simulink model "quat_difference"  (R2024a)
settings: Solver=VariableStepAuto  StartTime=0.0  StopTime=10.0  RelTol=1e-3
libraries: sharedtransform x5, aerolibutil x1
settings Model: Creator=bemran  LastModifiedBy=bemran

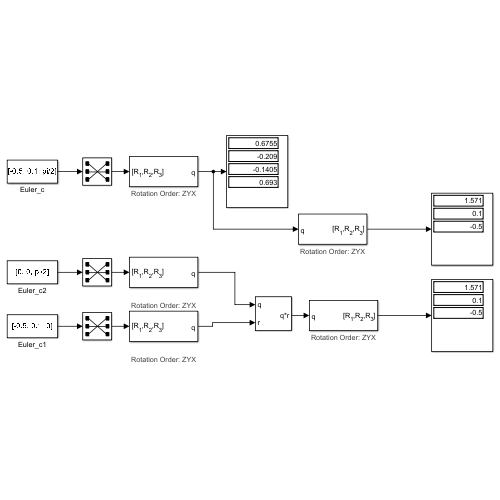
[thumbnail: Simulink's stored preview of the top-level diagram]
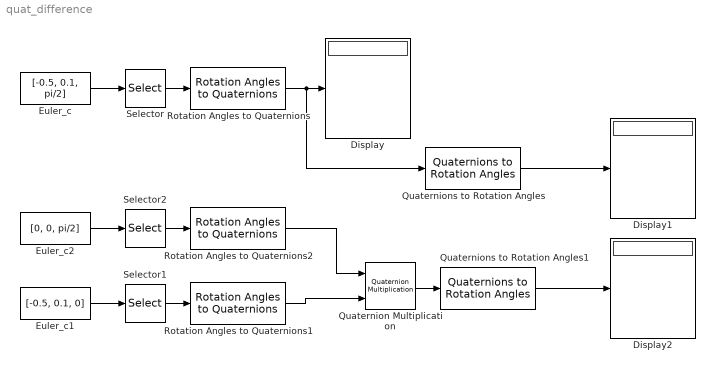
== system quat_difference ==
  Display : Display
  Display1 : Display
  Display2 : Display
  Euler_c : Constant  Value=[-0.5, 0.1, pi/2]
  Euler_c1 : Constant  Value=[-0.5, 0.1, 0]
  Euler_c2 : Constant  Value=[0, 0, pi/2]
  Quaternion Multiplication : aerolibutil/Quaternion Multiplication
  Quaternions to Rotation Angles : sharedtransform/Quaternions to Rotation Angles  rotationOrder=ZYX  aMode=aMode
  Quaternions to Rotation Angles1 : sharedtransform/Quaternions to Rotation Angles  rotationOrder=ZYX  aMode=aMode
  Rotation Angles to Quaternions : sharedtransform/Rotation Angles to Quaternions  rotationOrder=ZYX  aMode=aMode
  Rotation Angles to Quaternions1 : sharedtransform/Rotation Angles to Quaternions  rotationOrder=ZYX  aMode=aMode
  Rotation Angles to Quaternions2 : sharedtransform/Rotation Angles to Quaternions  rotationOrder=ZYX  aMode=aMode
  Selector : Selector  InputPortWidth=3  IndexOptions=Index vector (dialog)  Indices=[3 2 1]  OutputSizes=1
  Selector1 : Selector  InputPortWidth=3  IndexOptions=Index vector (dialog)  Indices=[3 2 1]  OutputSizes=1
  Selector2 : Selector  InputPortWidth=3  IndexOptions=Index vector (dialog)  Indices=[3 2 1]  OutputSizes=1
  wires:
  Selector/1 -> Rotation Angles to Quaternions/1
  Euler_c/1 -> Selector/1
  Rotation Angles to Quaternions/1 -> Quaternions to Rotation Angles/1, Display/1
  Euler_c1/1 -> Selector1/1
  Selector1/1 -> Rotation Angles to Quaternions1/1
  Selector2/1 -> Rotation Angles to Quaternions2/1
  Euler_c2/1 -> Selector2/1
  Rotation Angles to Quaternions1/1 -> Quaternion Multiplication/2
  Rotation Angles to Quaternions2/1 -> Quaternion Multiplication/1
  Quaternions to Rotation Angles/1 -> Display1/1
  Quaternion Multiplication/1 -> Quaternions to Rotation Angles1/1
  Quaternions to Rotation Angles1/1 -> Display2/1
